simulink model "s12_euler_ssprk3_muscl_minmod_ref"  (R2026a)
settings: Solver=FixedStepDiscrete  StopTime=0  FixedStep=1
model workspace (MAT data in the model file):
  S12_RK3_CFL = Simulink.Parameter
  S12_RK3_CFL.Value = 0.45
  S12_RK3_CFL.Complexity = 'real'
  S12_RK3_CFL.Dimensions = [1 1]
  S12_RK3_CFL.Description = 'CFL stability factor.'
  S12_RK3_CFL.DataType = 'auto'
  S12_RK3_Dx = Simulink.Parameter
  S12_RK3_Dx.Value = 0.005
  S12_RK3_Dx.Complexity = 'real'
  S12_RK3_Dx.Dimensions = [1 1]
  S12_RK3_Dx.Description = 'Uniform cell width.'
  S12_RK3_Dx.DataType = 'auto'
  S12_RK3_EndTime = Simulink.Parameter
  S12_RK3_EndTime.Value = 0.2
  S12_RK3_EndTime.Complexity = 'real'
  S12_RK3_EndTime.Dimensions = [1 1]
  S12_RK3_EndTime.Description = 'Integration end time.'
  S12_RK3_EndTime.DataType = 'auto'
  S12_RK3_Gamma = Simulink.Parameter
  S12_RK3_Gamma.Value = 1.4
  S12_RK3_Gamma.Complexity = 'real'
  S12_RK3_Gamma.Dimensions = [1 1]
  S12_RK3_Gamma.Description = 'Ratio of specific heats.'
  S12_RK3_Gamma.DataType = 'auto'
  S12_RK3_MaxSteps = Simulink.Parameter
  S12_RK3_MaxSteps.Value = 10000
  S12_RK3_MaxSteps.Complexity = 'real'
  S12_RK3_MaxSteps.Dimensions = [1 1]
  S12_RK3_MaxSteps.Description = 'Maximum accepted SSP-RK3 steps.'
  S12_RK3_MaxSteps.DataType = 'auto'
  S12_RK3_State = Simulink.Parameter
  S12_RK3_State.Value = [1 0 2.5 1 0 2.5 1 0 2.5 1 0 2.5 ... (600 elements, 3x200)]
  S12_RK3_State.Complexity = 'real'
  S12_RK3_State.Dimensions = [3 200]
  S12_RK3_State.Description = 'Classic Sod conservative state [rho; rho*u; rho*E], 3x200.'
  S12_RK3_State.DataType = 'auto'
settings Model: Creator=Jovi  LastModifiedBy=Jovi

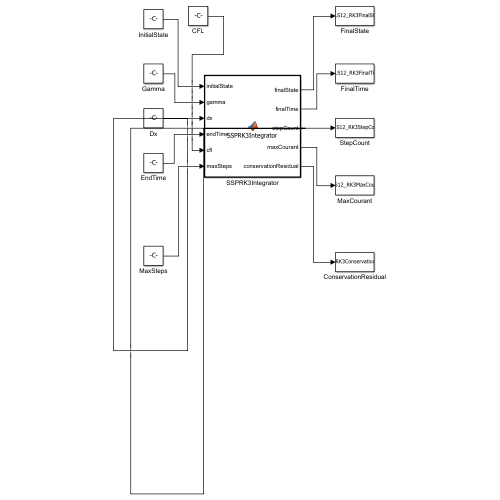
[thumbnail: Simulink's stored preview of the top-level diagram]
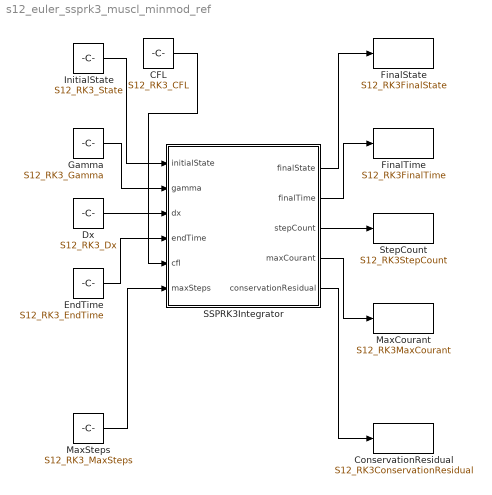
== system s12_euler_ssprk3_muscl_minmod_ref ==
  CFL : Constant  Value=S12_RK3_CFL
  ConservationResidual : ToWorkspace  VariableName=S12_RK3ConservationResidual  SampleTime=-1
  Dx : Constant  Value=S12_RK3_Dx
  EndTime : Constant  Value=S12_RK3_EndTime
  FinalState : ToWorkspace  VariableName=S12_RK3FinalState  SampleTime=-1
  FinalTime : ToWorkspace  VariableName=S12_RK3FinalTime  SampleTime=-1
  Gamma : Constant  Value=S12_RK3_Gamma
  InitialState : Constant  Value=S12_RK3_State
  MaxCourant : ToWorkspace  VariableName=S12_RK3MaxCourant  SampleTime=-1
  MaxSteps : Constant  Value=S12_RK3_MaxSteps
  SSPRK3Integrator : MATLAB Function  TreatAsAtomicUnit=on
  StepCount : ToWorkspace  VariableName=S12_RK3StepCount  SampleTime=-1
  wires:
  InitialState/1 -> SSPRK3Integrator/1(initialState)
  Gamma/1 -> SSPRK3Integrator/2(gamma)
  Dx/1 -> SSPRK3Integrator/3(dx)
  EndTime/1 -> SSPRK3Integrator/4(endTime)
  CFL/1 -> SSPRK3Integrator/5(cfl)
  MaxSteps/1 -> SSPRK3Integrator/6(maxSteps)
  SSPRK3Integrator/1(finalState) -> FinalState/1
  SSPRK3Integrator/2(finalTime) -> FinalTime/1
  SSPRK3Integrator/3(stepCount) -> StepCount/1
  SSPRK3Integrator/4(maxCourant) -> MaxCourant/1
  SSPRK3Integrator/5(conservationResidual) -> ConservationResidual/1

== matlab function s12_euler_ssprk3_muscl_minmod_ref/SSPRK3Integrator ==
  data: initialState input; finalState output; gamma input; dx input; endTime input; cfl input; maxSteps input; finalTime output; stepCount output; maxCourant output; conservationResidual output
function [finalState,finalTime,stepCount,maxCourant,conservationResidual] = SSPRK3Integrator(initialState,gamma,dx,endTime,cfl,maxSteps)
%SSPRK3INTEGRATOR Integrate the one-dimensional conservative Euler equations.
U = initialState;
time = 0.0;
stepCount = 0.0;
maxCourant = 0.0;
boundaryIntegral = zeros(3,1);

if ~(isfinite(gamma) && gamma > 1.0 && isfinite(dx) && dx > 0.0 && ...
        isfinite(endTime) && endTime >= 0.0 && isfinite(cfl) && cfl > 0.0 && ...
        isfinite(maxSteps) && maxSteps >= 0.0)
    error('S12:SSPRK3:InvalidInput','Invalid SSP-RK3 integration input.');
end
validateState(U,gamma);

while time < endTime
    if stepCount >= maxSteps
        error('S12:SSPRK3:MaxSteps','SSP-RK3 exhausted maxSteps before endTime.');
    end

    [rho,velocity,pressure] = recoverPrimitives(U,gamma);
    signalSpeed = max(abs(velocity) + sqrt(gamma*pressure./rho));
    if ~(isfinite(signalSpeed) && signalSpeed > 0.0)
        error('S12:SSPRK3:SignalSpeed','SSP-RK3 encountered an invalid signal speed.');
    end
    dt = min(cfl*dx/signalSpeed,endTime-time);
    if ~(isfinite(dt) && dt > 0.0)
        error('S12:SSPRK3:TimeStep','SSP-RK3 encountered an invalid time step.');
    end

    [L0,left0,right0] = spatialOperator(U,gamma,dx);
    U1 = U + dt*L0;
    [L1,left1,right1] = spatialOperator(U1,gamma,dx);
    U2 = 0.75*U + 0.25*(U1 + dt*L1);
    [L2,left2,right2] = spatialOperator(U2,gamma,dx);
    U = (1.0/3.0)*U + (2.0/3.0)*(U2 + dt*L2);

    boundaryIntegral = boundaryIntegral + dt*( ...
        (right0-left0)/6.0 + (right1-left1)/6.0 + ...
        2.0*(right2-left2)/3.0);

    validateState(U,gamma);
    stepCount = stepCount + 1.0;
    time = time + dt;
    maxCourant = max(maxCourant,dt*signalSpeed/dx);
end

if time ~= endTime
    error('S12:SSPRK3:EndTime','SSP-RK3 did not terminate exactly at endTime.');
end

finalState = U;
finalTime = time;
conservationResidual = ( ...
    dx*sum(finalState-initialState,2) + boundaryIntegral).';
end

function validateState(U,gamma)
if any(~isfinite(U(:)))
    error('S12:SSPRK3:NonfiniteState','SSP-RK3 encountered a nonfinite state.');
end
[rho,~,pressure] = recoverPrimitives(U,gamma);
if any(rho <= 0.0) || any(pressure <= 0.0)
    error('S12:SSPRK3:NonphysicalState','SSP-RK3 encountered a nonpositive density or pressure.');
end
end

function [rho,velocity,pressure] = recoverPrimitives(U,gamma)
rho = U(1,:);
velocity = U(2,:)./rho;
pressure = (gamma-1.0)*(U(3,:) - 0.5*rho.*velocity.^2);
end

function flux = physicalFlux(U,gamma)
[rho,velocity,pressure] = recoverPrimitives(U,gamma);
flux = [rho.*velocity; rho.*velocity.^2 + pressure; ...
    velocity.*(U(3,:) + pressure)];
end

function flux = hllcFlux(UL,UR,gamma)
[rhoL,uL,pL] = recoverPrimitives(UL,gamma);
[rhoR,uR,pR] = recoverPrimitives(UR,gamma);
aL = sqrt(gamma*pL/rhoL);
aR = sqrt(gamma*pR/rhoR);
sL = min(uL-aL,uR-aR);
sR = max(uL+aL,uR+aR);
sStar = (pR-pL + rhoL*uL*(sL-uL) - rhoR*uR*(sR-uR)) / ...
    (rhoL*(sL-uL) - rhoR*(sR-uR));

FL = physicalFlux(UL,gamma);
FR = physicalFlux(UR,gamma);
rhoStarL = rhoL*(sL-uL)/(sL-sStar);
rhoStarR = rhoR*(sR-uR)/(sR-sStar);
energyStarL = UL(3)/rhoL + (sStar-uL)*( ...
    sStar + pL/(rhoL*(sL-uL)));
energyStarR = UR(3)/rhoR + (sStar-uR)*( ...
    sStar + pR/(rhoR*(sR-uR)));
UStarL = rhoStarL*[1.0; sStar; energyStarL];
UStarR = rhoStarR*[1.0; sStar; energyStarR];

if 0.0 <= sL
    flux = FL;
elseif sL <= 0.0 && 0.0 <= sStar
    flux = FL + sL*(UStarL-UL);
elseif sStar <= 0.0 && 0.0 <= sR
    flux = FR + sR*(UStarR-UR);
else
    flux = FR;
end
end

function [rhs,leftFlux,rightFlux] = spatialOperator(U,gamma,dx)
cellCount = size(U,2);
interfaceFlux = zeros(3,cellCount+1);
[rho,velocity,pressure] = recoverPrimitives(U,gamma);
slopeRho = minmodSlopes(rho,false);
slopeVelocity = minmodSlopes(velocity,false);
slopePressure = minmodSlopes(pressure,false);
interfaceFlux(:,1) = hllcFlux(U(:,1),U(:,1),gamma);
for interfaceIndex = 1:(cellCount-1)
    rightIndex = interfaceIndex + 1;
    leftState = conservativeFromPrimitives(rho(interfaceIndex) + 0.5*slopeRho(interfaceIndex),velocity(interfaceIndex) + 0.5*slopeVelocity(interfaceIndex),pressure(interfaceIndex) + 0.5*slopePressure(interfaceIndex),gamma);
    rightState = conservativeFromPrimitives(rho(rightIndex) - 0.5*slopeRho(rightIndex),velocity(rightIndex) - 0.5*slopeVelocity(rightIndex),pressure(rightIndex) - 0.5*slopePressure(rightIndex),gamma);
    interfaceFlux(:,interfaceIndex+1) = hllcFlux(leftState,rightState,gamma);
end
interfaceFlux(:,cellCount+1) = hllcFlux(U(:,cellCount),U(:,cellCount),gamma);
rhs = zeros(size(U));
for cellIndex = 1:cellCount
    rhs(:,cellIndex) = -(interfaceFlux(:,cellIndex+1) - interfaceFlux(:,cellIndex))/dx;
end
leftFlux = physicalFlux(U(:,1),gamma);
rightFlux = physicalFlux(U(:,cellCount),gamma);
end

function U = conservativeFromPrimitives(rho,velocity,pressure,gamma)
U = [rho; rho.*velocity; pressure/(gamma-1.0) + 0.5*rho.*velocity.^2];
end

function slopes = minmodSlopes(values,isPeriodic)
cellCount = numel(values);
slopes = zeros(size(values));
if cellCount < 3
    return
end
if isPeriodic
    for cellIndex = 1:cellCount
        leftIndex = cellIndex - 1;
        if leftIndex < 1
            leftIndex = cellCount;
        end
        rightIndex = cellIndex + 1;
        if rightIndex > cellCount
            rightIndex = 1;
        end
        slopes(cellIndex) = minmod(values(cellIndex)-values(leftIndex),values(rightIndex)-values(cellIndex));
    end
else
    for cellIndex = 2:(cellCount-1)
        slopes(cellIndex) = minmod(values(cellIndex)-values(cellIndex-1),values(cellIndex+1)-values(cellIndex));
    end
end
end

function value = minmod(leftDelta,rightDelta)
if leftDelta*rightDelta <= 0.0
    value = 0.0;
elseif abs(leftDelta) <= abs(rightDelta)
    value = leftDelta;
else
    value = rightDelta;
end
end
